simulink model "Subsystem"  (R2020b)
settings: Solver=FixedStepAuto  StartTime=0.0  StopTime=10.0  FixedStep=1  RelTol=1e-3
settings Model: Creator=Varun  LastModifiedBy=Varun
settings DataIOCC: SaveOutput=off  SaveTime=off

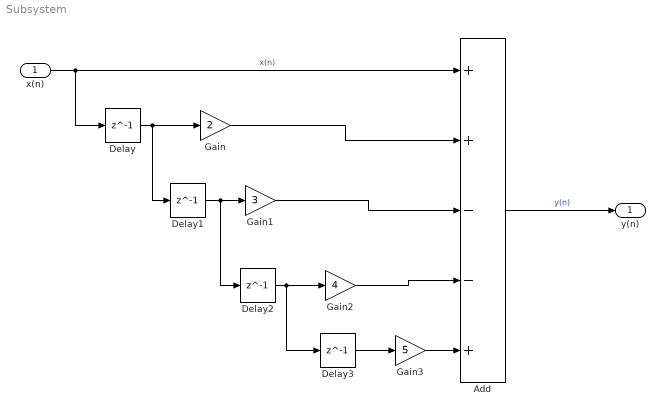
== system Subsystem ==
  x(n) : Inport  OutDataTypeStr=double  PortDimensions=1  SampleTime=[1,0]
  Add : Sum  Inputs=++--+
  Delay{,1..3} (4 alike) : Delay  DelayLength=1
  Gain : Gain  Gain=2
  Gain1 : Gain  Gain=3
  Gain2 : Gain  Gain=4
  Gain3 : Gain  Gain=5
  y(n) : Outport  OutDataTypeStr=double  PortDimensions=1  SampleTime=[1,0]
  wires:
  Delay3/1 -> Gain3/1
  Gain3/1 -> Add/5
  x(n)/1 -> Add/1, Delay/1  "x(n)"
  Delay2/1 -> Gain2/1, Delay3/1
  Delay/1 -> Gain/1, Delay1/1
  Gain2/1 -> Add/4
  Gain1/1 -> Add/3
  Delay1/1 -> Gain1/1, Delay2/1
  Gain/1 -> Add/2
  Add/1 -> y(n)/1  "y(n)"
